simulink model "wv_control_loop"  (R2018b)
settings: Solver=VariableStepAuto  StartTime=0.0  StopTime=20  RelTol=1e-3
values from neighbouring files (symbols this model uses):
  alpha = 0.2    [regbot_mg.m]
  Kp_wv = 7.756    [regbot_mg.m]
undefined symbols (not defined in the file or in its folder): denom_wv, num_wv, T_d, T_i
settings Model: Creator=megam  LastModifiedBy=megam

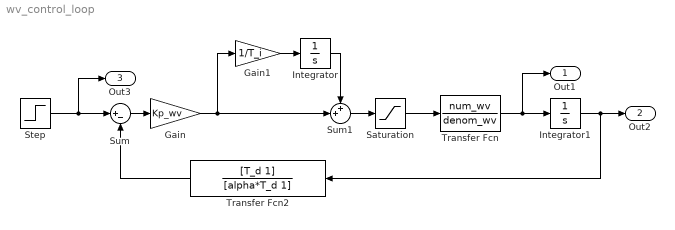
== system wv_control_loop ==
  Gain : Gain  Gain=Kp_wv
  Gain1 : Gain  Gain=1/T_i
  Integrator : Integrator  LimitOutput=on  UpperSaturationLimit=+3  LowerSaturationLimit=-3
  Integrator1 : Integrator
  Saturation : Saturate  UpperLimit=+3  LowerLimit=-3
  Step : Step  Time=0  After=0.5  SampleTime=0
  Sum : Sum  Inputs=|+-
  Sum1 : Sum  Inputs=++|
  Transfer Fcn : TransferFcn  Numerator=num_wv  Denominator=denom_wv
  Transfer Fcn2 : TransferFcn  Numerator=[T_d 1]  Denominator=[alpha*T_d 1]
  Out1 : Outport  SignalName=Velocity
  Out2 : Outport  Port=2  SignalName=Position
  Out3 : Outport  Port=3  SignalName=Position ref
  wires:
  Step/1 -> Out3/1, Sum/1
  Transfer Fcn/1 -> Out1/1, Integrator1/1
  Sum/1 -> Gain/1
  Gain/1 -> Gain1/1, Sum1/2
  Gain1/1 -> Integrator/1
  Integrator/1 -> Sum1/1
  Integrator1/1 -> Transfer Fcn2/1, Out2/1
  Transfer Fcn2/1 -> Sum/2
  Sum1/1 -> Saturation/1
  Saturation/1 -> Transfer Fcn/1
